simulink model "pid_inverse_pendulum"  (R2016b)
settings: Solver=VariableStepAuto  StartTime=0.0  StopTime=20  RelTol=1e-3
values from neighbouring files (symbols this model uses):
  A = [0 0 1 0; 0 0 0 1; 0 (b*d)/(a*c-b^2) -(c*e)/(a*c-b^2) 0; 0 (a*d)/(a*c-b^2) -(b*e)/(a*c-b^2) 0]    [jaya_pid_rotational_inverse_pendulum.m]
  B = [0 0 c*f/(a*c-b^2) b*f/(a*c-b^2)]'    [jaya_pid_rotational_inverse_pendulum.m]
  C = [1 0 0 0; 0 1 0 0; 0 0 1 0; 0 0 0 1]    [jaya_pid_rotational_inverse_pendulum.m]
  D = [0; 0; 0; 0]    [jaya_pid_rotational_inverse_pendulum.m]
  D_alpha = jaya_table(i, 3)    [jaya_pid_rotational_inverse_pendulum.m]
  D_theta = jaya_table(i, 6)    [jaya_pid_rotational_inverse_pendulum.m]
  I_alpha = jaya_table(i, 2)    [jaya_pid_rotational_inverse_pendulum.m]
  I_theta = jaya_table(i, 5)    [jaya_pid_rotational_inverse_pendulum.m]
  P_alpha = jaya_table(i, 1)    [jaya_pid_rotational_inverse_pendulum.m]
  P_theta = jaya_table(i, 4)    [jaya_pid_rotational_inverse_pendulum.m]
libraries: simulink_extras x4, simulink x2
settings Model: Creator=Truc  LastModifiedBy=Truc

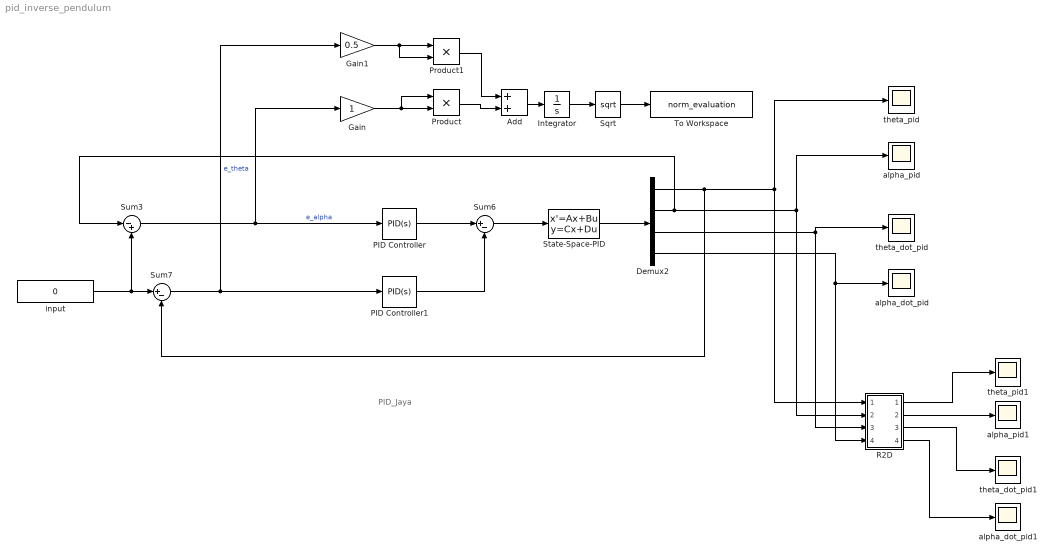
== system pid_inverse_pendulum ==
  note: PID_Jaya
  Add : Sum
  Demux2 : Demux
  Gain : Gain
  Gain1 : Gain  Gain=0.5
  Integrator : Integrator
  PID Controller : simulink/Continuous/PID Controller  Controller=PID  TimeDomain=Continuous-time  SampleTime=-1  IntegratorMethod=Forward Euler  FilterMethod=Forward Euler  Form=Parallel  UseFilter=on  ControllerParametersSource=internal  P=P_alpha  I=I_alpha  D=D_alpha  N=100  InitialConditionSource=internal  InitialConditionForIntegrator=0  InitialConditionForFilter=0  ExternalReset=none  LimitOutput=off  UpperSaturationLimit=inf  LowerSaturationLimit=-inf  LinearizeAsGain=on  AntiWindupMode=none  Kb=1  TrackingMode=off  Kt=1  PParamMin=[]  PParamMax=[]  IParamMin=[]  IParamMax=[]  DParamMin=[]  DParamMax=[]  NParamMin=[]  NParamMax=[]  KbParamMin=[]  KbParamMax=[]  KtParamMin=[]  KtParamMax=[]  POutMin=[]  POutMax=[]  IOutMin=[]  IOutMax=[]  DOutMin=[]  DOutMax=[]  NOutMin=[]  NOutMax=[]  KbOutMin=[]  KbOutMax=[]  KtOutMin=[]  KtOutMax=[]  IntegratorOutMin=[]  IntegratorOutMax=[]  FilterOutMin=[]  FilterOutMax=[]  SumOutMin=[]  SumOutMax=[]  SumI1OutMin=[]  SumI1OutMax=[]  SumI2OutMin=[]  SumI2OutMax=[]  SumI3OutMin=[]  SumI3OutMax=[]  SumDOutMin=[]  SumDOutMax=[]  SaturationOutMin=[]  SaturationOutMax=[]  IntegratorContinuousStateAttributes=''  IntegratorStateMustResolveToSignalObject=off  IntegratorRTWStateStorageClass=Auto  FilterContinuousStateAttributes=''  FilterStateMustResolveToSignalObject=off  FilterRTWStateStorageClass=Auto  DifferentiatorICPrevScaledInput=0  DifferentiatorOutMin=[]  DifferentiatorOutMax=[]
  PID Controller1 : simulink/Continuous/PID Controller  Controller=PID  TimeDomain=Continuous-time  SampleTime=-1  IntegratorMethod=Forward Euler  FilterMethod=Forward Euler  Form=Parallel  UseFilter=on  ControllerParametersSource=internal  P=P_theta  I=I_theta  D=D_theta  N=100  InitialConditionSource=internal  InitialConditionForIntegrator=0  InitialConditionForFilter=0  ExternalReset=none  LimitOutput=off  UpperSaturationLimit=inf  LowerSaturationLimit=-inf  LinearizeAsGain=on  AntiWindupMode=none  Kb=1  TrackingMode=off  Kt=1  PParamMin=[]  PParamMax=[]  IParamMin=[]  IParamMax=[]  DParamMin=[]  DParamMax=[]  NParamMin=[]  NParamMax=[]  KbParamMin=[]  KbParamMax=[]  KtParamMin=[]  KtParamMax=[]  POutMin=[]  POutMax=[]  IOutMin=[]  IOutMax=[]  DOutMin=[]  DOutMax=[]  NOutMin=[]  NOutMax=[]  KbOutMin=[]  KbOutMax=[]  KtOutMin=[]  KtOutMax=[]  IntegratorOutMin=[]  IntegratorOutMax=[]  FilterOutMin=[]  FilterOutMax=[]  SumOutMin=[]  SumOutMax=[]  SumI1OutMin=[]  SumI1OutMax=[]  SumI2OutMin=[]  SumI2OutMax=[]  SumI3OutMin=[]  SumI3OutMax=[]  SumDOutMin=[]  SumDOutMax=[]  SaturationOutMin=[]  SaturationOutMax=[]  IntegratorContinuousStateAttributes=''  IntegratorStateMustResolveToSignalObject=off  IntegratorRTWStateStorageClass=Auto  FilterContinuousStateAttributes=''  FilterStateMustResolveToSignalObject=off  FilterRTWStateStorageClass=Auto  DifferentiatorICPrevScaledInput=0  DifferentiatorOutMin=[]  DifferentiatorOutMax=[]
  Product : Product
  Product1 : Product
  R2D : Subsystem
  Sqrt : Sqrt  SaturateOnIntegerOverflow=on
  State-Space-PID : StateSpace  A=A  B=B  C=C  D=D  X0=[4 4 0 0]*pi/180
  Sum3 : Sum  Inputs=|-+
  Sum6 : Sum  Inputs=|+-
  Sum7 : Sum  Inputs=|+-
  To Workspace : ToWorkspace  VariableName=norm_evaluation  SaveFormat=Timeseries  SampleTime=-1
      settings: MaxDataPoints=1
  alpha_dot_pid : Scope
  alpha_dot_pid1 : Scope
  alpha_pid : Scope
  alpha_pid1 : Scope
  input : Constant  Value=0
  theta_dot_pid : Scope
  theta_dot_pid1 : Scope
  theta_pid : Scope
  theta_pid1 : Scope
  wires:
  R2D/1(Out1) -> theta_pid1/1
  R2D/2(Out2) -> alpha_pid1/1
  R2D/3(Out3) -> theta_dot_pid1/1
  R2D/4(Out4) -> alpha_dot_pid1/1
  Demux2/4 -> R2D/4(In4), alpha_dot_pid/1
  Demux2/3 -> R2D/3(In3), theta_dot_pid/1
  Demux2/1 -> Sum7/2, R2D/1(In1), theta_pid/1
  Demux2/2 -> Sum3/1, R2D/2(In2), alpha_pid/1
  State-Space-PID/1 -> Demux2/1
  Sum6/1 -> State-Space-PID/1
  input/1 -> Sum3/2, Sum7/1
  PID Controller1/1 -> Sum6/2
  PID Controller/1 -> Sum6/1
  Integrator/1 -> Sqrt/1
  Sqrt/1 -> To Workspace/1
  Product1/1 -> Add/1
  Add/1 -> Integrator/1
  Product/1 -> Add/2
  Gain/1 -> Product/1, Product/2
  Sum3/1 -> Gain/1, PID Controller/1  "e_alpha"
  Sum7/1 -> PID Controller1/1, Gain1/1  "e_theta"
  Gain1/1 -> Product1/2, Product1/1

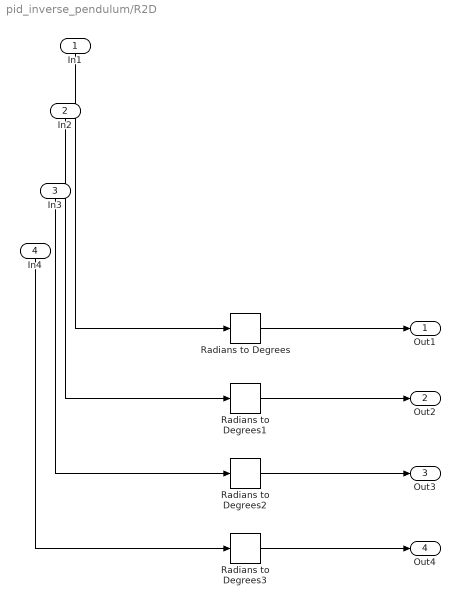
== system pid_inverse_pendulum/R2D ==
  In1 : Inport
  In2 : Inport  Port=2
  In3 : Inport  Port=3
  In4 : Inport  Port=4
  Radians to Degrees{,1..3} (4 alike) : simulink_extras/Transformations/Radians to Degrees
  Out1 : Outport
  Out2 : Outport  Port=2
  Out3 : Outport  Port=3
  Out4 : Outport  Port=4
  wires:
  Radians to Degrees/1 -> Out1/1
  Radians to Degrees1/1 -> Out2/1
  Radians to Degrees3/1 -> Out4/1
  Radians to Degrees2/1 -> Out3/1
  In4/1 -> Radians to Degrees3/1
  In3/1 -> Radians to Degrees2/1
  In1/1 -> Radians to Degrees/1
  In2/1 -> Radians to Degrees1/1
